simulink model "PGA_MPC_MODEL"  (R2024b)
settings: Solver=ode4  StartTime=0.0  StopTime=180  FixedStep=0.0005  RelTol=1e-3
values from neighbouring files (symbols this model uses):
  Road_Curvature_Map = [Global_S, Global_K]    [Road_Condition_Info.m]
  Road_Mu_Map = [Global_S, Global_Mu]    [Road_Condition_Info.m]
  Target_Speed_Map = [Global_S, Global_Vx]    [Road_Condition_Info.m]
undefined symbols (not defined in the file or in its folder): MotorData, Sim_Mu_Set, Sim_Vx_Set
libraries: Solver_SF x1
(part 2 of 3)

== matlab function PGA_MPC_MODEL/Subsystem1/MATLAB Function17 ==
  data: Vx input; r_d output; delta_f input; mu input; m input; lf input; lr input; K_s output; r_ideal output; Kf0 input; Kr0 input; g input; r_limit output
function [r_d, K_s, r_ideal, r_limit] = ReferenceYawRate(Vx, delta_f, mu, m, lf, lr, Kf0, Kr0, g)
% =========================================================================
% 参考横摆角速度生成 (鲁棒增强版)
% 修复内容：低速奇点保护、物理极限柔性化、输出平滑
% =========================================================================

    % 1. 参数默认值与保护
    if nargin < 9, g = 9.81; end
    
    % 输入数据维度清洗 (强制转为标量 double)
    Vx_in = double(Vx(1));
    delta_in = double(delta_f(1));
    mu_in = double(mu(1));

    % 速度方向与绝对值处理
    Vx_sign = sign(Vx_in);
    if Vx_sign == 0, Vx_sign = 1; end
    Vx_abs = abs(Vx_in);
    
    % 基础防除零保护 (计算模型用)
    Vx_safe = max(Vx_abs, 0.5); 

    % =====================================================================
    % 2. 计算稳态增益 (Steady State Gain)
    % =====================================================================
    K_s = m / (2 * (lf + lr)^2) * (lr/Kf0 - lf/Kr0);

    % =====================================================================
    % 3. 计算理想横摆角速度 (Linear 2DOF Model)
    % =====================================================================
    % 分母：1 + K * V^2
    denom = (lf + lr) * (1 + K_s * Vx_safe^2);
    
    if abs(denom) < 0.1
        r_ideal = 0;
    else
        % r_ideal = (Vx / L(1+KV^2)) * delta
        r_ideal = (Vx_safe / denom) * delta_in * Vx_sign; 
    end

    % =====================================================================
    % 4. 计算物理极限 (【关键修复点】)
    % =====================================================================
    % 原公式：Limit = 0.85 * mu * g / Vx
    % 问题：当车辆甩尾速度掉到 1m/s 时，Limit 会变成 0.85*0.8*9.8/1 = 6.6 rad/s (380度/秒)
    % 修复：计算极限时，假设速度至少为 5m/s (虚拟速度钳位)
    % 逻辑：低速时侧向加速度其实达不到 mu*g，因为离心力不够，所以这样限制更符合物理
    
    Vx_for_limit = max(Vx_abs, 5.0); 
    
    % 计算理论上限
    r_limit_val = 0.85 * mu_in * g / Vx_for_limit;
    
    % 【双重保险】增加一个绝对硬限幅 (例如 1.5 rad/s ≈ 85 deg/s)
    % 防止任何情况下的数值爆炸
    r_limit_val = min(r_limit_val, 1.5);

    % =====================================================================
    % 5. 柔性限幅 (Saturation)
    % =====================================================================
    if r_ideal > r_limit_val
        r_d_raw = r_limit_val;
    elseif r_ideal < -r_limit_val
        r_d_raw = -r_limit_val;
    else
        r_d_raw = r_ideal;
    end

    % =====================================================================
    % 6. 强力滤波 (平滑输出)
    % =====================================================================
    persistent rd_prev
    if isempty(rd_prev), rd_prev = 0; end
    
    % 滤波系数：0.05 代表非常强的滤波 (响应慢，但稳)，如果觉得滞后太大可改为 0.1
    alpha_filter = 0.05; 
    
    r_d_smooth = (1 - alpha_filter) * rd_prev + alpha_filter * r_d_raw;
    
    % 更新记忆
    rd_prev = r_d_smooth;

    % =====================================================================
    % 7. 输出类型转换
    % =====================================================================
    r_d = double(r_d_smooth);
    r_ideal = double(r_ideal);
    r_limit = double(r_limit_val);
    
end

== matlab function PGA_MPC_MODEL/Subsystem1/MATLAB Function15 ==
  data: Vx_cmd input; Vx_act_raw input; T_total output; Ax_cmd input; m input; g input; r_e input; Kp input; Ki input; dt input; is_reset input; T_ff output; T_fb output; delta_steering input; Mu_in input; Curv_in input; Beta_in input; SI_in input
function [T_total, T_ff, T_fb] = Calc_Total_Demand_Torque( ...
    Vx_cmd, Vx_act_raw, Ax_cmd, ...
    m, g, r_e, ...
    Kp, Ki, dt, is_reset, delta_steering, Mu_in, ...
    Curv_in, Beta_in, SI_in)
%#codegen
% =========================================================================
% Upper-layer nominal total torque generator v2
% 适配你的 H-MPC / AD-MPC 版本
%
% 核心原则：
%   1. 只负责生成“名义总需求转矩”
%   2. 不根据 Mu / Curv / Beta / SI 主动降扭
%   3. 不抢下层 MPC 的 Wsum 自适应调度功能
%   4. 自动处理 Vx_cmd 是 km/h 还是 m/s 的问题
%
% 推荐外部参数：
%   Kp = 12
%   Ki = 0.3
%   dt = 0.01
% =========================================================================

    persistent Vx_f I_term T_prev

    % =========================================================
    % 0. reset and basic protection
    % =========================================================
    reset_flag = false;
    if double(is_reset(1)) > 0.5
        reset_flag = true;
    end

    if dt <= 1e-6
        dt = 0.01;
    end

    Vx_cmd_raw = double(Vx_cmd(1));
    Vx_act_raw_use = double(Vx_act_raw(1));
    Ax_cmd_use = double(Ax_cmd(1));

    % =========================================================
    % 1. speed unit auto-detection
    % =========================================================
    % 你的工况是 68 km/h，CarSim Vx 通常约 18.9 m/s。
    % 如果输入大于 40，基本可以判断是 km/h，自动除以 3.6。
    if abs(Vx_cmd_raw) > 40.0
        Vx_cmd_use = Vx_cmd_raw / 3.6;
    else
        Vx_cmd_use = Vx_cmd_raw;
    end

    if abs(Vx_act_raw_use) > 40.0
        Vx_act_use = Vx_act_raw_use / 3.6;
    else
        Vx_act_use = Vx_act_raw_use;
    end

    Vx_cmd_use = max(0.0, Vx_cmd_use);
    Vx_act_use = max(0.0, Vx_act_use);

    if isempty(Vx_f) || reset_flag
        Vx_f   = Vx_act_use;
        I_term = 0.0;
        T_prev = 0.0;
    end

    % =========================================================
    % 2. actual speed filtering
    % =========================================================
    alpha_v = 0.15;
    Vx_f = (1.0 - alpha_v) * Vx_f + alpha_v * Vx_act_use;
    Vx_act = Vx_f;

    % =========================================================
    % 3. physical feedforward torque
    % =========================================================
    Cd = 0.30;
    Af = 2.8;
    rho = 1.206;
    f_roll = 0.015;

    Vx_ff = Vx_act;

    if abs(Vx_ff) > 0.2
        sgn_v = sign(Vx_ff);
    else
        sgn_v = 0.0;
    end

    % 不让 Ax_cmd 把上层变成激进加速器
    Ax_cmd_use = min(max(Ax_cmd_use, -0.8), 0.8);

    F_aero = 0.5 * rho * Cd * Af * Vx_ff * Vx_ff * sgn_v;
    F_roll = m * g * f_roll * sgn_v;
    F_acc  = m * Ax_cmd_use;

    T_ff = (F_aero + F_roll + F_acc) * r_e;

    % =========================================================
    % 4. mild PI speed feedback
    % =========================================================
    e_v = Vx_cmd_use - Vx_act;

    deadband = 0.08;

    if e_v > deadband
        e_eff = e_v - deadband;
    elseif e_v < -deadband
        e_eff = e_v + deadband;
    else
        e_eff = 0.0;
    end

    % 防止外部参数给太大
    Kp_eff = min(max(double(Kp), 0.0), 18.0);
    Ki_eff = min(max(double(Ki), 0.0), 1.0);

    P_term = Kp_eff * e_eff;

    % =========================================================
    % 5. integral with anti-windup
    % =========================================================
    I_max = 70.0;
    I_min = -90.0;

    I_candidate = I_term + Ki_eff * e_eff * dt;
    I_candidate = min(max(I_candidate, I_min), I_max);

    T_candidate = T_ff + P_term + I_candidate;

    % 名义总转矩保护，不根据风险变，只做物理合理范围限制
    T_max_limit = 320.0;
    T_min_limit = -180.0;

    if (T_candidate > T_max_limit && e_eff > 0.0)
        % 上限饱和且还想继续加速，不积分
    elseif (T_candidate < T_min_limit && e_eff < 0.0)
        % 下限饱和且还想继续减速，不积分
    else
        I_term = I_candidate;
    end

    T_cmd = T_ff + P_term + I_term;

    % =========================================================
    % 6. overspeed protection
    % =========================================================
    % 这不是稳定性控制，只是基本速度闭环保护：
    % 实际速度超过目标时，不允许上层继续大正转矩。
    over_v = Vx_act - Vx_cmd_use;

    if over_v > 0.25
        T_overspeed_limit = T_ff - 70.0 * over_v;
        T_cmd = min(T_cmd, T_overspeed_limit);
    end

    T_cmd = min(max(T_cmd, T_min_limit), T_max_limit);

    % =========================================================
    % 7. torque rate limit
    % =========================================================
    % 只做执行器平滑，不用风险信号。
    dT_up_rate = 350.0;    % Nm/s
    dT_dn_rate = 650.0;    % Nm/s

    dT_up = dT_up_rate * dt;
    dT_dn = dT_dn_rate * dt;

    if reset_flag
        T_total = T_cmd;
        T_prev = T_total;
    else
        dT = T_cmd - T_prev;

        if dT > dT_up
            T_total = T_prev + dT_up;
        elseif dT < -dT_dn
            T_total = T_prev - dT_dn;
        else
            T_total = T_cmd;
        end

        T_prev = T_total;
    end

    T_fb = T_total - T_ff;

    T_total = double(T_total);
    T_ff    = double(T_ff);
    T_fb    = double(T_fb);

end

== matlab function PGA_MPC_MODEL/Subsystem1/MATLAB Function18 ==
  settings: updateMethod=DISCRETE  sampleTime=0.01
  data: Vx_target_input input; Vx_safe_cmd output; dt input; Ax_cmd_final output
function [Vx_safe_cmd, Ax_cmd_final] = Constant_Speed_Planner(Vx_target_input, dt)
    % Constant_Speed_Planner
    % 功能：生成恒定目标车速和加速度指令
    
    % ================= 1. 数据预处理 (维度安全锁) =================
    % 强制转换为 double
    temp_v = double(Vx_target_input);
    
    % 【关键修改】防止输入变成向量 [4x1]
    % 如果输入是向量，取第一个元素或取平均值，确保输出是标量 [1x1]
    if numel(temp_v) > 1
        target_v = mean(temp_v); % 或者 target_v = temp_v(1);
    else
        target_v = temp_v;
    end
    
    % 限幅保护
    if isnan(target_v)
        target_v = 0;
    end
    target_v = max(target_v, 0); 

    % ================= 2. 指令生成 =================
    Vx_safe_cmd = target_v;
    
    % 理论加速度设为0
    Ax_cmd_final = 0; 
    
    % (可选) 如果未来想用 dt 做平滑处理，可以在这里写逻辑
    % 目前 dt 虽然未被使用，但保留在输入端口没问题，不会报错
end

== matlab function PGA_MPC_MODEL/Subsystem1/MATLAB Function19 ==
  data: Vx input; Beta input; Beta_dot input; mu input; SI_Out output
function SI_Out = fcn_Calculate_SI(Vx, Beta, Beta_dot, mu)
%#codegen
% =========================================================================
% SI calculation module without upper saturation
% Purpose:
%   Used for post-processing, logging, and quantitative comparison.
%   The upper bound of 1.5 is removed so that the true instability severity
%   can be observed in simulation results.
% =========================================================================

    %% 1. Input processing
    v_in = max(abs(double(Vx(1))), 1.0);
    beta_in = double(Beta(1));
    beta_dot_in = double(Beta_dot(1));
    mu_in = max(min(double(mu(1)), 0.9), 0.2);

    %% 2. Phase-plane boundary slope
    % Slope = -0.000005 * v^2 + 0.003898 * v + 0.022393
    Slope = -0.000005 * v_in^2 + 0.003898 * v_in + 0.022393;

    %% 3. Stability boundary Blim
    e1 = -0.038102; 
    e2 =  0.195963; 
    e3 =  0.005132;
    e4 =  0.235299; 
    e5 = -0.011306; 
    e6 = -0.000252;
    e7 = -0.013729; 
    e8 =  0.000720; 
    e9 = -0.000046;

    Blim = e1 + ...
           e2 * mu_in + e3 * v_in + ...
           e4 * mu_in^2 + e5 * mu_in * v_in + e6 * v_in^2 + ...
           e7 * mu_in^2 * v_in + e8 * mu_in * v_in^2 + ...
           e9 * mu_in^2 * v_in^2;

    % Boundary protection
    if Blim < 0.001
        Blim = 0.001;
    end

    %% 4. SI calculation
    % Stability boundary:
    % | beta + Slope * beta_dot | <= Blim
    Phase_Val = beta_in + Slope * beta_dot_in;
    SI_phase = abs(Phase_Val) / abs(Blim);

    %% 5. Physical fallback
    % If sideslip angle exceeds about 10 deg, the vehicle is regarded as
    % approaching severe instability.
    SI_Phys = abs(beta_in) / 0.17;

    %% 6. Final SI output without upper saturation
    SI_Out = max(SI_phase, SI_Phys);

    % Keep only the lower bound protection. No upper saturation is applied.
    SI_Out = max(SI_Out, 0);
end

== matlab function PGA_MPC_MODEL/Subsystem1/MATLAB Function23 ==
  data: Fy_fl input; Cf_eq output; Fy_fr input; Fy_rl input; Fy_rr input; Alpha_fl input; Alpha_fr input; Alpha_rl input; Alpha_rr input; Cf0 input; Cr0 input; Cr_eq output; Mu_Current input
function [Cf_eq, Cr_eq] = fcn_Calc_Equivalent_Stiffness_Filtered(...
    Fy_fl, Fy_fr, Fy_rl, Fy_rr, ...
    Alpha_fl, Alpha_fr, Alpha_rl, Alpha_rr, ...
    Cf0, Cr0, Mu_Current) % ★ 新增输入: 当前路面附着 Mu_Current
% =========================================================================
% 非线性侧偏刚度估算模块 (前馈预警 + 实时估算混合版)
% =========================================================================
    persistent Cf_prev Cr_prev
    if isempty(Cf_prev)
        Cf_prev = Cf0 * 2; 
        Cr_prev = Cr0 * 2;
    end
    
    % =====================================================================
    % ★ 核心新增：基于附着系数的前馈压制 (Feed-forward Penalty) ★
    % 当车进入冰雪路面时，不用等侧滑发生，直接从物理极限上压低标称刚度！
    % =====================================================================
    mu_nominal = 0.85;
    mu_real = max(min(double(Mu_Current(1)), 1.0), 0.1);
    % 计算附着衰减系数
    mu_ratio = mu_real / mu_nominal; 
    
    % 前馈修正后的基础刚度 (冰面上基础刚度会瞬间掉下来)
    Cf_base_dyn = (Cf0 * 2) * mu_ratio;
    Cr_base_dyn = (Cr0 * 2) * mu_ratio;

    Fy_front_sum = abs(Fy_fl + Fy_fr);
    Fy_rear_sum  = abs(Fy_rl + Fy_rr);
    Alpha_front_avg = abs(Alpha_fl + Alpha_fr) / 2.0;
    Alpha_rear_avg  = abs(Alpha_rl + Alpha_rr) / 2.0;
    
    alpha_deadzone = 0.0087; 
    
    if Alpha_front_avg > alpha_deadzone
        Cf_inst = Fy_front_sum / Alpha_front_avg;
    else
        Cf_inst = Cf_base_dyn; % 小角度时用前馈修正的刚度
    end
    
    if Alpha_rear_avg > alpha_deadzone
        Cr_inst = Fy_rear_sum / Alpha_rear_avg;
    else
        Cr_inst = Cr_base_dyn; % 小角度时用前馈修正的刚度
    end
    
    % ★ 限幅逻辑也要跟着附着系数前馈一起下降 ★
    Cf_min = Cf_base_dyn * 0.3;  Cf_max = Cf_base_dyn * 1.5;
    Cr_min = Cr_base_dyn * 0.3;  Cr_max = Cr_base_dyn * 1.5;
    
    Cf_target = max(min(Cf_inst, Cf_max), Cf_min);
    Cr_target = max(min(Cr_inst, Cr_max), Cr_min);
    
    % 为了应对附着突变，如果是从高附着到低附着（刚度需要暴降），加快滤波速度
    if Cf_target < Cf_prev
        lambda = 0.3; % 变滑了，降刚度要快！(0.05太慢了)
    else
        lambda = 0.05; % 恢复抓地力，慢慢升
    end
    
    Cf_filt = (1 - lambda) * Cf_prev + lambda * Cf_target;
    Cr_filt = (1 - lambda) * Cr_prev + lambda * Cr_target;
    
    Cf_prev = Cf_filt; Cr_prev = Cr_filt;
    Cf_eq = Cf_filt; Cr_eq = Cr_filt;
end

== matlab function PGA_MPC_MODEL/Subsystem1/MATLAB Function5 ==
  data: Vx input; Sx_fr output; Vy input; r input; omega_fr input; delta_f input; lf input; twf input; Re input; Sy_fr output; Vsx_fr output; Vsy_fr output
function [Sx_fr, Sy_fr, Vsx_fr, Vsy_fr] = Cal_UniTire_FullData_FR(Vx, Vy, r, omega_fr, delta_f, lf, twf, Re)
% Cal_UniTire_FullData_FR - 右前轮全参数计算

    % === 1. 运动学解算 ===
    % 右前轮：纵向 +lf, 横向 -twf/2 (右侧)
    % Vx修正: 右侧轮在左转(r>0)时线速度增加，所以是 + r*(twf/2)
    V_cx = Vx + r * (twf / 2);  
    V_cy = Vy + r * lf;         

    % === 2. 坐标旋转 (车轮坐标系) ===
    cos_d = cos(delta_f);
    sin_d = sin(delta_f);
    
    V_long = V_cx * cos_d + V_cy * sin_d;
    V_lat  = -V_cx * sin_d + V_cy * cos_d;

    % === 3. 计算滑移速度 (能耗用) ===
    V_wheel = omega_fr * Re;
    Vsx_fr = V_wheel - V_long; % 纵向滑移速度
    Vsy_fr = V_lat;            % 侧向滑移速度

    % === 4. 计算滑移率 (轮胎模型用) ===
    V_long_safe = max(abs(V_long), 1.0); 
    
    Sx_fr = Vsx_fr / V_long_safe;
    Sy_fr = -Vsy_fr / V_long_safe; % UniTire定义带负号

    % === 5. 限幅 ===
    Sx_fr = max(min(Sx_fr, 1.5), -1.5);
    Sy_fr = max(min(Sy_fr, 1.5), -1.5);
end

== matlab function PGA_MPC_MODEL/Subsystem1/MATLAB Function6 ==
  data: Vx input; Sx_rl output; Vy input; r input; omega_rl input; lr input; twr input; Re input; Sy_rl output; Vsx_rl output; Vsy_rl output
function [Sx_rl, Sy_rl, Vsx_rl, Vsy_rl] = Cal_UniTire_FullData_RL(Vx, Vy, r, omega_rl, lr, twr, Re)
% Cal_UniTire_FullData_RL - 左后轮全参数计算
% 注意：后轮默认无转向角 (delta = 0)

    % === 1. 运动学解算 ===
    % 左后轮：纵向 -lr, 横向 +twr/2 (左侧)
    % Vcx: 左侧减去横摆分量
    % Vcy: 后轴减去横摆分量 (Vy - r*lr)
    V_cx = Vx - r * (twr / 2);  
    V_cy = Vy - r * lr;         

    % === 2. 坐标旋转 (后轮 delta=0) ===
    % cos(0)=1, sin(0)=0，其实就是不用旋转
    V_long = V_cx;
    V_lat  = V_cy;

    % === 3. 计算滑移速度 (能耗用) ===
    V_wheel = omega_rl * Re;
    Vsx_rl = V_wheel - V_long; 
    Vsy_rl = V_lat;            

    % === 4. 计算滑移率 (轮胎模型用) ===
    V_long_safe = max(abs(V_long), 1.0); 
    
    Sx_rl = Vsx_rl / V_long_safe;
    Sy_rl = -Vsy_rl / V_long_safe;

    % === 5. 限幅 ===
    Sx_rl = max(min(Sx_rl, 1.5), -1.5);
    Sy_rl = max(min(Sy_rl, 1.5), -1.5);
end

== matlab function PGA_MPC_MODEL/Subsystem1/MATLAB Function7 ==
  data: Vx input; Sx_rr output; Vy input; r input; omega_rr input; lr input; twr input; Re input; Sy_rr output; Vsx_rr output; Vsy_rr output
function [Sx_rr, Sy_rr, Vsx_rr, Vsy_rr] = Cal_UniTire_FullData_RR(Vx, Vy, r, omega_rr, lr, twr, Re)
% Cal_UniTire_FullData_RR - 右后轮全参数计算
% 注意：后轮默认无转向角 (delta = 0)

    % === 1. 运动学解算 ===
    % 右后轮：纵向 -lr, 横向 -twr/2 (右侧)
    % Vcx: 右侧加上横摆分量
    % Vcy: 后轴减去横摆分量
    V_cx = Vx + r * (twr / 2);  
    V_cy = Vy - r * lr;         

    % === 2. 坐标旋转 (后轮 delta=0) ===
    V_long = V_cx;
    V_lat  = V_cy;

    % === 3. 计算滑移速度 (能耗用) ===
    V_wheel = omega_rr * Re;
    Vsx_rr = V_wheel - V_long; 
    Vsy_rr = V_lat;            

    % === 4. 计算滑移率 (轮胎模型用) ===
    V_long_safe = max(abs(V_long), 1.0); 
    
    Sx_rr = Vsx_rr / V_long_safe;
    Sy_rr = -Vsy_rr / V_long_safe;

    % === 5. 限幅 ===
    Sx_rr = max(min(Sx_rr, 1.5), -1.5);
    Sy_rr = max(min(Sy_rr, 1.5), -1.5);
end

== matlab function PGA_MPC_MODEL/Subsystem1/unitire轮胎力 ==
  data: Vx input; Vy input; r input; Sx_fl output; omega_fl input; delta_f input; lf input; twf input; Sy_fl output; Re input; Vsx_fl output; Vsy_fl output
function [Sx_fl, Sy_fl, Vsx_fl, Vsy_fl] = Cal_UniTire_FullData_FL(Vx, Vy, r, omega_fl, delta_f, lf, twf, Re)
% Cal_UniTire_FullData_FL - 左前轮全参数计算
% 输出: 
%   Sx, Sy: UniTire定义的滑移率 (无量纲) -> 用于查表或公式算力
%   Vsx, Vsy: 轮胎接地点滑移速度 (m/s) -> 用于 P = F * V 算能耗

    % === 1. 运动学解算：计算【轮心】在【车身坐标系】下的速度 ===
    % (左前轮：纵向 +lf, 横向 +twf/2)
    % 注意：横摆 r 对纵向速度的影响是 -r*y, 对横向速度的影响是 +r*x
    V_cx = Vx - r * (twf / 2);  
    V_cy = Vy + r * lf;         

    % === 2. 坐标旋转：转换到【车轮坐标系】 ===
    cos_d = cos(delta_f);
    sin_d = sin(delta_f);
    
    % V_long: 车轮滚动方向速度 (即纵向速度 Vx_wheel)
    % V_lat:  车轮侧向速度 (即侧向速度 Vy_wheel)
    V_long = V_cx * cos_d + V_cy * sin_d;
    V_lat  = -V_cx * sin_d + V_cy * cos_d;

    % === 3. 计算滑移速度 (能耗计算的核心) ===
    % 轮缘线速度
    V_wheel = omega_fl * Re;

    % 纵向滑移速度 (Vsx): 也就是大家常说的“滑移速度差”
    % 物理含义：轮胎接地点相对于地面的向后速度
    Vsx_fl = V_wheel - V_long; 

    % 侧向滑移速度 (Vsy): 
    % 物理含义：轮胎整体侧滑的速度
    Vsy_fl = V_lat; 

    % === 4. 计算滑移率 (UniTire 轮胎力模型的核心) ===
    % 分母保护：防止停车或低速时除零，导致仿真崩溃
    % 选取 max(abs(V_long), 1.0) 是为了在低速下保证数值稳定
    V_long_safe = max(abs(V_long), 1.0); 
    
    % --- 纵向滑移率 Sx ---
    % UniTire 定义: Sx = (V_wheel - V_long) / V_long
    % 等价于: Sx = Vsx / V_long
    Sx_fl = Vsx_fl / V_long_safe;

    % --- 侧向滑移率 Sy ---
    % UniTire 定义: Sy = - V_lat / V_long
    % 等价于: Sy = - Vsy / V_long
    % 注意：UniTire 的 Sy 定义通常带有负号 (对应 -tan(alpha))
    Sy_fl = -Vsy_fl / V_long_safe;

    % === 5. 物理限幅 (防止数值爆炸) ===
    % 仅对滑移率限幅，滑移速度(Vsx/Vsy)是物理真值，不要限幅！
    Sx_fl = max(min(Sx_fl, 1.5), -1.5);
    Sy_fl = max(min(Sy_fl, 1.5), -1.5);

end

== matlab function PGA_MPC_MODEL/Subsystem1/侧偏角计算 ==
  data: Vx input; alpha_fl output; Vy input; r input; delta_f_rad input; lf input; lr input; twf input; twr input; alpha_fr output; alpha_rl output; alpha_rr output
function [alpha_fl, alpha_fr, alpha_rl, alpha_rr] = Block2_SlipAngle(...
    Vx, Vy, r, delta_f_rad, lf, lr, twf, twr)
% =========================================================================
% BLOCK2_SLIPANGLE - 四轮侧偏角计算 (纯弧度版)
% 
% [关键设置]
% 1. 输入 delta_f_rad 必须是【弧度】(您已在外部转换好)。
% 2. 输出 alpha 均为【弧度】。
% 3. 符号修正：采用 (转向角 - 速度角) 逻辑，确保左转产生正滑移角。
% =========================================================================

    % 1. 速度方向保护 (防止分母为0)
    Vx_safe = max(abs(Vx), 0.1) * sign(Vx); 
    if Vx_safe == 0, Vx_safe = 0.1; end
    
    % 2. 轮心速度解算 (运动学公式)
    % -----------------------------------------------------------
    % 左前轮 (Left-Front)
    Vx_fl = Vx_safe - (r * twf) / 2;
    Vy_fl = Vy + (r * lf);
    
    % 右前轮 (Right-Front)
    Vx_fr = Vx_safe + (r * twf) / 2;
    Vy_fr = Vy + (r * lf);
    
    % 左后轮 (Left-Rear)
    Vx_rl = Vx_safe - (r * twr) / 2;
    Vy_rl = Vy - (r * lr);
    
    % 右后轮 (Right-Rear)
    Vx_rr = Vx_safe + (r * twr) / 2;
    Vy_rr = Vy - (r * lr);
    
    % 3. 侧偏角计算 (核心修正)
    % -----------------------------------------------------------
    % 公式：Alpha = 转向角 - 速度矢量角
    % atan2 计算结果天然是弧度，与您的输入 delta_f_rad (弧度) 直接相减
    
    % 左前
    theta_fl = atan2(Vy_fl, Vx_fl);
    alpha_fl = delta_f_rad - theta_fl; 
    
    % 右前
    theta_fr = atan2(Vy_fr, Vx_fr);
    alpha_fr = delta_f_rad - theta_fr;
    
    % 左后 (后轮转向角 delta = 0)
    theta_rl = atan2(Vy_rl, Vx_rl);
    alpha_rl = 0 - theta_rl; 
    
    % 右后
    theta_rr = atan2(Vy_rr, Vx_rr);
    alpha_rr = 0 - theta_rr; 

    % 4. 输出清理
    % -----------------------------------------------------------
    % 确保输出为实数
    alpha_fl = real(alpha_fl);
    alpha_fr = real(alpha_fr);
    alpha_rl = real(alpha_rl);
    alpha_rr = real(alpha_rr);
    
    % [注意] 输出的是弧度！
    % 如果接下来的刚度模块或轮胎模块需要弧度，直接连线即可。
    % 后面【千万不要】再接那个 pi/180 的 Gain 模块了！
end

== matlab function PGA_MPC_MODEL/Subsystem1/横纵向附着系数 ==
  data: road_condition input; mu_x output; slip_ratio input; mu_y output
function [mu_x, mu_y] = FrictionCoefficientLookup(road_condition, slip_ratio)
% 基于路面条件和滑移率的摩擦系数查表
% 输入: road_condition - 路面类型 (1=冰面, 2=雪面, 3=湿沥青, 4=干沥青)
%       slip_ratio - 当前滑移率（可选，用于动态调整）

    switch road_condition
        case 1 % 冰面（论文实验条件）
            mu_x = 0.2;
            mu_y = 0.18;  % 横向摩擦系数通常略低
            
        case 2 % 雪面
            mu_x = 0.3;
            mu_y = 0.25;
            
        case 3 % 湿沥青
            mu_x = 0.5;
            mu_y = 0.45;
            
        case 4 % 干沥青
            mu_x = 0.85;
            mu_y = 0.80;
            
        otherwise
            mu_x = 0.8;
            mu_y = 0.75;
    end
    
    % 可选：基于滑移率的动态调整（Burckhardt模型简化版）
    if nargin > 1
        % 典型摩擦系数-滑移率曲线（冰面）
        if road_condition == 1
            optimal_slip = 0.08;  % 冰面最佳滑移率
            if slip_ratio > optimal_slip
                % 超过最佳滑移率后摩擦系数下降
                mu_x = mu_x * (1 - 0.5 * (slip_ratio - optimal_slip));
                mu_y = mu_y * (1 - 0.6 * (slip_ratio - optimal_slip));
            end
        end
    end
end

== matlab function PGA_MPC_MODEL/Subsystem1/MATLAB Function1 ==
  data: Sx_fl input; Sy_fl input; Fx_fl output; Fz_fl input; mu_x input; mu_y input; Kx input; Ky input; Fy_fl output; Fbar_x_fl output; Fbar_y_fl output; E input
function [Fx_fl, Fy_fl, Fbar_x_fl, Fbar_y_fl] = Cal_Force_FL(Sx_fl, Sy_fl, Fz_fl, mu_x, mu_y, Kx, Ky, E)
% Cal_Force_FL - 左前轮 UniTire (完整版)
% 输入:
% Sx_fl, Sy_fl: 纵横向滑移率
% Fz_fl: 垂向载荷 (N)
% mu_x, mu_y: 纵向/横向 峰值附着系数 (例如 1.0, 0.9)
% Kx, Ky: 轮胎纵向/横向刚度 (N/1)
% E: UniTire 曲率因子 (通常 0.5~1.0，决定峰值后的形状)

% 0. 数据保护
Fz_safe = max(Fz_fl, 100); % 防止 Fz=0 报错
% 1. 计算相对滑移率 (Relative Slip, phi)
% 分别针对纵向和横向极限进行归一化
% phi_x = (Kx * Sx) / (mu_x * Fz)
phi_x = (Kx * abs(Sx_fl)) / (mu_x * Fz_safe);
phi_y = (Ky * abs(Sy_fl)) / (mu_y * Fz_safe);
% 合成相对滑移率 (摩擦椭圆耦合核心)
phi = sqrt(phi_x^2 + phi_y^2);

% 2. 计算总归一化力 (F_bar)
% UniTire 经验公式: F_bar = 1 - exp(-phi - E * phi^2)
% 这里的 E 就是您要找回的曲率因子
if phi < 1e-6
F_bar = 0;
else
F_bar = 1 - exp(-phi - E * phi^2);
end

% 3. 分解回横纵向 (分配方向)
% Fbar_x 是归一化分量 (0~1)
if phi < 1e-6
Fbar_x_fl = 0;
Fbar_y_fl = 0;
else
Fbar_x_fl = F_bar * (phi_x / phi);
Fbar_y_fl = F_bar * (phi_y / phi);
end

% 4. 计算真实物理力 (Physical Force, N)
% 必须乘回各自方向的极限力 (mu * Fz)
Max_Force_X = mu_x * Fz_safe;
Max_Force_Y = mu_y * Fz_safe;
Fx_abs = Fbar_x_fl * Max_Force_X;
Fy_abs = Fbar_y_fl * Max_Force_Y;

% 5. 恢复符号
Fx_fl = sign(Sx_fl) * Fx_abs;
Fy_fl = sign(Sy_fl) * Fy_abs;
end

== matlab function PGA_MPC_MODEL/Subsystem1/MATLAB Function8 ==
  data: Sx_rl input; Sy_rl input; Fx_rl output; Fz_rl input; mu_x input; mu_y input; Kx input; Ky input; Fy_rl output; Fbar_x_rl output; Fbar_y_rl output; E input

function [Fx_rl, Fy_rl, Fbar_x_rl, Fbar_y_rl] = Cal_Force_RL(Sx_rl, Sy_rl, Fz_rl, mu_x, mu_y, Kx, Ky, E)
% Cal_Force_RL - 左后轮 UniTire (完整版)

Fz_safe = max(Fz_rl, 100);

% 1. 相对滑移率
phi_x = (Kx * abs(Sx_rl)) / (mu_x * Fz_safe);
phi_y = (Ky * abs(Sy_rl)) / (mu_y * Fz_safe);
phi = sqrt(phi_x^2 + phi_y^2);

% 2. 总归一化力
if phi < 1e-6
F_bar = 0;
else
F_bar = 1 - exp(-phi - E * phi^2);
end

% 3. 分量分配
if phi < 1e-6
Fbar_x_rl = 0;
Fbar_y_rl = 0;
else
Fbar_x_rl = F_bar * (phi_x / phi);
Fbar_y_rl = F_bar * (phi_y / phi);
end

% 4. 真实力
Fx_rl = sign(Sx_rl) * (Fbar_x_rl * (mu_x * Fz_safe));
Fy_rl = sign(Sy_rl) * (Fbar_y_rl * (mu_y * Fz_safe));
end

== matlab function PGA_MPC_MODEL/Subsystem1/MATLAB Function9 ==
  data: Sx_fr input; Sy_fr input; Fx_fr output; Fz_fr input; mu_x input; mu_y input; Kx input; Ky input; Fy_fr output; Fbar_x_fr output; Fbar_y_fr output; E input
function [Fx_fr, Fy_fr, Fbar_x_fr, Fbar_y_fr] = Cal_Force_FR(Sx_fr, Sy_fr, Fz_fr, mu_x, mu_y, Kx, Ky, E)
% Cal_Force_FR - 右前轮 UniTire (完整版)

Fz_safe = max(Fz_fr, 100);

% 1. 相对滑移率
phi_x = (Kx * abs(Sx_fr)) / (mu_x * Fz_safe);
phi_y = (Ky * abs(Sy_fr)) / (mu_y * Fz_safe);
phi = sqrt(phi_x^2 + phi_y^2);

% 2. 总归一化力 (带 E)
if phi < 1e-6
F_bar = 0;
else
F_bar = 1 - exp(-phi - E * phi^2);
end

% 3. 分量分配
if phi < 1e-6
Fbar_x_fr = 0;
Fbar_y_fr = 0;
else
Fbar_x_fr = F_bar * (phi_x / phi);
Fbar_y_fr = F_bar * (phi_y / phi);
end

% 4. 真实力 (乘回 mu*Fz)
Fx_fr = sign(Sx_fr) * (Fbar_x_fr * (mu_x * Fz_safe));
Fy_fr = sign(Sy_fr) * (Fbar_y_fr * (mu_y * Fz_safe));
end

== matlab function PGA_MPC_MODEL/Subsystem1/MATLAB Function10 ==
  data: Sx_rr input; Sy_rr input; Fx_rr output; Fz_rr input; mu_x input; mu_y input; Kx input; Ky input; E input; Fy_rr output; Fbar_x_rr output; Fbar_y_rr output
function [Fx_rr, Fy_rr, Fbar_x_rr, Fbar_y_rr] = Cal_Force_RR(Sx_rr, Sy_rr, Fz_rr, mu_x, mu_y, Kx, Ky, E)
% Cal_Force_RR - 右后轮 UniTire (完整版)

Fz_safe = max(Fz_rr, 100);

% 1. 相对滑移率
phi_x = (Kx * abs(Sx_rr)) / (mu_x * Fz_safe);
phi_y = (Ky * abs(Sy_rr)) / (mu_y * Fz_safe);
phi = sqrt(phi_x^2 + phi_y^2);

% 2. 总归一化力
if phi < 1e-6
F_bar = 0;
else
F_bar = 1 - exp(-phi - E * phi^2);
end

% 3. 分量分配
if phi < 1e-6
Fbar_x_rr = 0;
Fbar_y_rr = 0;
else
Fbar_x_rr = F_bar * (phi_x / phi);
Fbar_y_rr = F_bar * (phi_y / phi);
end

% 4. 真实力
Fx_rr = sign(Sx_rr) * (Fbar_x_rr * (mu_x * Fz_safe));
Fy_rr = sign(Sy_rr) * (Fbar_y_rr * (mu_y * Fz_safe));
end

== matlab function PGA_MPC_MODEL/Subsystem1/MATLAB Function14 ==
  data: NN_Weights output; Vx_kmh input; Vref_kmh input; Mu_current input; Kappa_current input; Mu_preview input; Kappa_preview input
function NN_Weights = Call_NN_Mapper(Vx_kmh, Vref_kmh, Mu_current, Kappa_current, Mu_preview, Kappa_preview)
%#codegen
% =========================================================================
% Reference-speed-aware risk-preserving 4D BO-BPNN weight mapper
%
% BPNN input:
%   X_NN = [V_NN, mu_risk, kappa_risk, D_safe]^T
%
% Key idea:
%   1) The BPNN still uses a 4D input.
%   2) The first input is not the raw measured speed, but a risk-preserving
%      speed feature V_NN.
%   3) In low-risk conditions, V_NN follows the measured speed Vx.
%   4) In high-risk conditions, V_NN approaches the reference-speed-aware
%      risk speed, but is capped to avoid excessive conservativeness.
% =========================================================================

    NN_Weights = zeros(5, 1, 'double');

    %% ============================================================
    % 0. Tunable parameters
    % ============================================================
    Ts_ctrl = 0.01;          % Control sampling time, s

    D_low  = 0.50;           % Risk-gate lower threshold
    D_high = 0.70;           % Risk-gate upper threshold

    DeltaV_cap = 10.0;        % km/h, max allowed gap between V_NN and Vx
                             % If SI is still high, try 10~12.
                             % If speed drops too much, try 5~6.

    lambda_D = 0.10;         % 1/s, linear decay rate of D_safe

    %% ============================================================
    % 1. Signal reading and protection
    % ============================================================
    Vx = double(Vx_kmh(1));
    if ~isfinite(Vx)
        Vx = 60.0;
    end
    Vx = min(max(Vx, 0.0), 120.0);

    Vref = double(Vref_kmh(1));
    if ~isfinite(Vref) || Vref <= 1.0
        Vref = Vx;
    end
    Vref = min(max(Vref, 0.0), 120.0);

    Mu_c = double(Mu_current(1));
    Mu_p = double(Mu_preview(1));

    if ~isfinite(Mu_c) || Mu_c <= 0
        Mu_c = 0.85;
    end

    if ~isfinite(Mu_p) || Mu_p <= 0
        Mu_p = Mu_c;
    end

    mu_risk = min(Mu_c, Mu_p);
    mu_risk = max(mu_risk, 0.10);

    Kappa_c = abs(double(Kappa_current(1)));
    Kappa_p = abs(double(Kappa_preview(1)));

    if ~isfinite(Kappa_c)
        Kappa_c = 0.0;
    end

    if ~isfinite(Kappa_p)
        Kappa_p = 0.0;
    end

    kappa_risk = max(Kappa_c, Kappa_p);

    %% ============================================================
    % 2. Reference-speed-aware risk gate
    % ============================================================
    D_ref = ((Vref / 3.6)^2 * kappa_risk) / max(mu_risk * 9.81, 1e-6);
    D_ref = min(max(D_ref, 0.0), 1.0);

    gamma = (D_ref - D_low) / max(D_high - D_low, 1e-6);
    gamma = min(max(gamma, 0.0), 1.0);

    %% ============================================================
    % 3. Risk-preserving speed feature
    % ============================================================
    V_risk = min(Vref, Vx + DeltaV_cap);
    V_risk = max(V_risk, Vx);

    V_NN = (1.0 - gamma) * Vx + gamma * V_risk;
    V_NN = min(max(V_NN, 0.0), 120.0);

    %% ============================================================
    % 4. Risk calculation with linear peak-hold decay
    % ============================================================
    D_raw = ((V_NN / 3.6)^2 * kappa_risk) / max(mu_risk * 9.81, 1e-6);
    D_raw = min(max(D_raw, 0.0), 1.0);

    persistent D_safe_prev;
    if isempty(D_safe_prev)
        D_safe_prev = 0.0;
    end

    D_safe = max(D_raw, D_safe_prev - lambda_D * Ts_ctrl);
    D_safe = min(max(D_safe, 0.0), 1.0);
    D_safe_prev = D_safe;

    %% ============================================================
    % 5. BPNN forward inference
    % ============================================================
    X_in = [V_NN; mu_risk; kappa_risk; D_safe];

    NN_out = BPNN_Core_Ultimate_Res(X_in);

    %% ============================================================
    % 6. Physical baseline and NN residual reconstruction
    % ============================================================
    base_R = 4.5 - 3.5 * D_safe;
    base_W = 1.0 + 3.5 * D_safe;

    res_R_alloc = max(-2.0, min(2.0, NN_out(3)));
    res_W_slip  = max(-2.0, min(3.0, NN_out(5)));

    log_R_alloc_nn = base_R + res_R_alloc;
    log_W_slip_nn  = base_W + res_W_slip;

    log_Q_beta_nn = NN_out(1);
    log_Q_yaw_nn  = NN_out(2);
    log_R_rate_nn = NN_out(4) - 0.5 * (D_safe^2);

    %% ============================================================
    % 7. Risk-dependent safety envelope for W_slip
    % ============================================================
    envelope_W = -16.2 * (D_safe^2) + 32.8 * D_safe - 11.6;
    envelope_W = max(0.0, envelope_W);

    log_W_slip_final = max(log_W_slip_nn, envelope_W);

    %% ============================================================
    % 8. High-risk priority shift
    % ============================================================
    risk_barrier = max(0.0, D_safe - 0.7) / 0.3;
    risk_barrier = min(max(risk_barrier, 0.0), 1.0);

    penalty_others = 1.0 * risk_barrier;

    log_R_alloc_final = log_R_alloc_nn - penalty_others;
    log_R_rate_final  = log_R_rate_nn  - penalty_others;
    log_Q_beta_final  = log_Q_beta_nn  - penalty_others;
    log_Q_yaw_final   = log_Q_yaw_nn   - penalty_others;

    %% ============================================================
    % 9. Log-domain bounds
    % ============================================================
    log_W_slip_final  = max(-1.0, min(5.5, log_W_slip_final));
    log_R_alloc_final = max(-1.0, min(6.0, log_R_alloc_final));
    log_R_rate_final  = max(-1.0, min(6.0, log_R_rate_final));
    log_Q_beta_final  = max(-1.0, min(6.0, log_Q_beta_final));
    log_Q_yaw_final   = max(-1.0, min(6.0, log_Q_yaw_final));

    %% ============================================================
    % 10. Log-domain filtering
    % ============================================================
    logW_raw = [
        log_Q_beta_final;
        log_Q_yaw_final;
        log_R_alloc_final;
        log_R_rate_final;
        log_W_slip_final
    ];

    persistent logW_prev;
    if isempty(logW_prev)
        logW_prev = logW_raw;
    end

    alpha = 0.1 + 0.3 * D_safe;
    alpha = min(max(alpha, 0.05), 0.45);

    logW_filt = (1.0 - alpha) * logW_prev + alpha * logW_raw;
    logW_prev = logW_filt;

    %% ============================================================
    % 11. Exponential reconstruction
    % ============================================================
    NN_Weights(1) = 10^logW_filt(1);   % Q_beta
    NN_Weights(2) = 10^logW_filt(2);   % Q_r
    NN_Weights(3) = 10^logW_filt(3);   % R_alloc
    NN_Weights(4) = 10^logW_filt(4);   % R_rate
    NN_Weights(5) = 10^logW_filt(5);   % W_slip
end

== matlab function PGA_MPC_MODEL/Subsystem1/MATLAB Function16 ==
  data: Fx_fl input; Px_fl output; Fy_fl input; Sx_fl input; Sy_fl input; Vx input; Vy input; r input; delta_f input; lf input; twf input; Py_fl output
function [Px_fl, Py_fl] = Cal_Power_FL(Fx_fl, Fy_fl, Sx_fl, Sy_fl, Vx, Vy, r, delta_f, lf, twf)
% Cal_Power_FL - 左前轮横纵向滑移功耗计算
% 基于 UniTire 模型定义的滑移率和力进行能量损耗计算
%
% 输入:
%   Fx_fl, Fy_fl: 轮胎纵向/横向力 (N) [来自力计算模块]
%   Sx_fl, Sy_fl: 轮胎纵向/横向滑移率 [来自滑移率模块]
%   Vx, Vy: 质心速度 (m/s)
%   r: 横摆角速度 (rad/s)
%   delta_f: 前轮转角 (rad)
%   lf: 质心到前轴距离 (m)
%   twf: 前轮距 (m)
%
% 输出:
%   Px_fl: 纵向滑移功耗 (W)
%   Py_fl: 横向滑移功耗 (W)

    % 1. 重新计算轮心纵向速度 V_long (用于将滑移率还原为滑移速度)
    % 运动学：左前轮位置 (+lf, +twf/2)
    V_cx = Vx - r * (twf / 2); % 减去横摆线速度
    V_cy = Vy + r * lf;        % 加上横摆线速度

    % 坐标旋转到车轮坐标系
    cos_d = cos(delta_f);
    sin_d = sin(delta_f);
    
    % V_long 是车轮滚动方向的速度
    V_long = V_cx * cos_d + V_cy * sin_d;
    
    % 保护：防止低速除零或噪声，与滑移率模块保持一致的基准
    V_long_abs = max(abs(V_long), 1.0);

    % 2. 计算纵向滑移功耗 (Longitudinal Slip Power)
    % 公式: Power = Force * Sliding_Velocity
    % Sliding_Velocity_X = Sx * V_long
    % 取绝对值因为功耗总是正值 (能量耗散)
    Px_fl = abs(Fx_fl * (Sx_fl * V_long_abs));

    % 3. 计算横向滑移功耗 (Lateral Slip Power)
    % 公式: Power = Force * Lateral_Sliding_Velocity
    % 根据 UniTire 定义: Sy = -V_lat / V_long  => V_lat = -Sy * V_long
    % 同样取绝对值
    Py_fl = abs(Fy_fl * (Sy_fl * V_long_abs));

end

== matlab function PGA_MPC_MODEL/Subsystem1/MATLAB Function21 ==
  data: Fx input; E_long_J output; E_lat_J output; Fy input; Vsx input; Vsy input; dt input; is_reset input; E_slip_J output; E_slip_kWh output; P_long_W output; P_lat_W output
function [E_long_J, E_lat_J, E_slip_J, E_slip_kWh, P_long_W, P_lat_W] = ...
    Cal_Slip_Energy_Internal_v2(Fx, Fy, Vsx, Vsy, dt, is_reset)
%#codegen
% =========================================================================
% Tire slip dissipation calculation
%
% Fx, Fy  : [4x1] tire longitudinal/lateral forces, N
% Vsx,Vsy : [4x1] longitudinal/lateral sliding velocities, m/s
% dt      : sample time, s
%
% E_long_J = integral(sum(|Fx .* Vsx|) dt)
% E_lat_J  = integral(sum(|Fy .* Vsy|) dt)
% =========================================================================

    persistent E_long_acc E_lat_acc

    if isempty(E_long_acc) || double(is_reset(1)) > 0.5
        E_long_acc = 0.0;
        E_lat_acc  = 0.0;
    end

    Fx_vec  = double(reshape(Fx,  4, 1));
    Fy_vec  = double(reshape(Fy,  4, 1));
    Vsx_vec = double(reshape(Vsx, 4, 1));
    Vsy_vec = double(reshape(Vsy, 4, 1));

    dt_in = double(dt(1));
    if isnan(dt_in) || isinf(dt_in) || dt_in <= 1e-6
        dt_in = 0.01;
    end

    for i = 1:4
        if isnan(Fx_vec(i)) || isinf(Fx_vec(i)), Fx_vec(i) = 0.0; end
        if isnan(Fy_vec(i)) || isinf(Fy_vec(i)), Fy_vec(i) = 0.0; end
        if isnan(Vsx_vec(i)) || isinf(Vsx_vec(i)), Vsx_vec(i) = 0.0; end
        if isnan(Vsy_vec(i)) || isinf(Vsy_vec(i)), Vsy_vec(i) = 0.0; end
    end

    P_long_W = sum(abs(Fx_vec .* Vsx_vec));
    P_lat_W  = sum(abs(Fy_vec .* Vsy_vec));

    E_long_acc = E_long_acc + P_long_W * dt_in;
    E_lat_acc  = E_lat_acc  + P_lat_W  * dt_in;

    E_long_J = E_long_acc;
    E_lat_J  = E_lat_acc;
    E_slip_J = E_long_acc + E_lat_acc;

    E_slip_kWh = E_slip_J / 3.6e6;
end

== matlab function PGA_MPC_MODEL/Subsystem1/MATLAB Function22 ==
  data: Fx_fr input; Px_fr output; Fy_fr input; Sx_fr input; Sy_fr input; Vx input; Vy input; r input; delta_f input; lf input; twf input; Py_fr output
function [Px_fr, Py_fr] = Cal_Power_FR(Fx_fr, Fy_fr, Sx_fr, Sy_fr, Vx, Vy, r, delta_f, lf, twf)
% Cal_Power_FR - 右前轮横纵向滑移功耗计算
% 注意：运动学计算中的符号与左轮不同

    % 1. 重新计算轮心纵向速度 V_long
    % 运动学：右前轮位置 (+lf, -twf/2 => 右侧通常定义为y轴负方向或正方向，此处依据您之前的代码逻辑)
    % 依据之前的逻辑：右轮横摆分量是 Vx + r*(twf/2)
    V_cx = Vx + r * (twf / 2); 
    V_cy = Vy + r * lf;

    % 坐标旋转
    cos_d = cos(delta_f);
    sin_d = sin(delta_f);
    
    V_long = V_cx * cos_d + V_cy * sin_d;
    V_long_abs = max(abs(V_long), 1.0);

    % 2. 纵向滑移功耗
    Px_fr = abs(Fx_fr * (Sx_fr * V_long_abs));

    % 3. 横向滑移功耗
    Py_fr = abs(Fy_fr * (Sy_fr * V_long_abs));

end

== matlab function PGA_MPC_MODEL/Subsystem1/MATLAB Function24 ==
  data: Fx_rl input; Px_rl output; Fy_rl input; Sx_rl input; Sy_rl input; Vx input; Vy input; r input; lr input; twr input; Py_rl output
function [Px_rl, Py_rl] = Cal_Power_RL(Fx_rl, Fy_rl, Sx_rl, Sy_rl, Vx, Vy, r, lr, twr)
% Cal_Power_RL - 左后轮横纵向滑移功耗计算
% 后轮无转向角 delta，故 V_long 直接等于 V_cx

    % 1. 重新计算轮心纵向速度 V_long
    % 运动学：左后轮位置 (-lr, +twr/2)
    % 左轮：Vx - r * (twr/2)
    V_long = Vx - r * (twr / 2);
    
    % 后轮无转向，无需坐标旋转，V_long 即为轮心纵向速度
    V_long_abs = max(abs(V_long), 1.0);

    % 2. 纵向滑移功耗
    Px_rl = abs(Fx_rl * (Sx_rl * V_long_abs));

    % 3. 横向滑移功耗
    Py_rl = abs(Fy_rl * (Sy_rl * V_long_abs));

end

== matlab function PGA_MPC_MODEL/Subsystem1/MATLAB Function25 ==
  data: Fx_rr input; Px_rr output; Fy_rr input; Sx_rr input; Sy_rr input; Vx input; Vy input; r input; lr input; twr input; Py_rr output
function [Px_rr, Py_rr] = Cal_Power_RR(Fx_rr, Fy_rr, Sx_rr, Sy_rr, Vx, Vy, r, lr, twr)
% Cal_Power_RR - 右后轮横纵向滑移功耗计算

    % 1. 重新计算轮心纵向速度 V_long
    % 运动学：右后轮位置 (-lr, -twr/2)
    % 右轮：Vx + r * (twr/2)
    V_long = Vx + r * (twr / 2);
    
    V_long_abs = max(abs(V_long), 1.0);

    % 2. 纵向滑移功耗
    Px_rr = abs(Fx_rr * (Sx_rr * V_long_abs));

    % 3. 横向滑移功耗
    Py_rr = abs(Fy_rr * (Sy_rr * V_long_abs));

end

== matlab function PGA_MPC_MODEL/Subsystem1/MATLAB Function26 ==
  data: Sx_vec input; Sx_abs_vec output; Fx_vec input; Fy_vec input; Fz_vec input; Mu_in input; Sx_max output; Sx_rms output; Eta_vec output; Eta_max output; Eta_rms output; Debug_Info output
function [Sx_abs_vec, Sx_max, Sx_rms, Eta_vec, Eta_max, Eta_rms, Debug_Info] = ...
    Calc_Slip_And_TireUtilization_Vec(Sx_vec, Fx_vec, Fy_vec, Fz_vec, Mu_in)
%#codegen
% =========================================================================
% Calc_Slip_And_TireUtilization_Vec
%
% 输入（推荐全部为 4x1 列向量）：
%   Sx_vec = [Sx_fl; Sx_fr; Sx_rl; Sx_rr]
%   Fx_vec = [Fx_fl; Fx_fr; Fx_rl; Fx_rr]
%   Fy_vec = [Fy_fl; Fy_fr; Fy_rl; Fy_rr]
%   Fz_vec = [Fz_fl; Fz_fr; Fz_rl; Fz_rr]
%   Mu_in  = 当前路面附着系数
%
% 输出：
%   Sx_abs_vec : 四轮绝对纵向滑移率 [4x1]
%   Sx_max     : 四轮最大绝对纵向滑移率
%   Sx_rms     : 四轮纵向滑移率 RMS
%   Eta_vec    : 四轮附着利用率 [4x1]
%   Eta_max    : 四轮最大附着利用率
%   Eta_rms    : 四轮附着利用率 RMS
%   Debug_Info : 调试输出 [6x1]
%
% 公式：
%   Sx_max(t) = max_i |Sx_i(t)|
%   Sx_rms(t) = sqrt( (1/4) * sum_i Sx_i(t)^2 )
%   Eta_i(t)  = sqrt( (Fx_i/(mu*Fz_i))^2 + (Fy_i/(mu*Fz_i))^2 )
% =========================================================================

%% 1) 输入整理与保护
% 强制转成 4x1 列向量（Simulink 中请把输入维度直接设成 [4 1]）
Sx = reshape(double(Sx_vec), 4, 1);
Fx = reshape(double(Fx_vec), 4, 1);
Fy = reshape(double(Fy_vec), 4, 1);
Fz = reshape(double(Fz_vec), 4, 1);

% NaN / Inf 保护
for i = 1:4
    if isnan(Sx(i)) || isinf(Sx(i))
        Sx(i) = 0.0;
    end
    if isnan(Fx(i)) || isinf(Fx(i))
        Fx(i) = 0.0;
    end
    if isnan(Fy(i)) || isinf(Fy(i))
        Fy(i) = 0.0;
    end
    if isnan(Fz(i)) || isinf(Fz(i))
        Fz(i) = 0.0;
    end
end

Mu_safe = double(Mu_in(1));
if isnan(Mu_safe) || isinf(Mu_safe)
    Mu_safe = 0.85;
end
Mu_safe = max(0.05, min(Mu_safe, 1.20));

% 垂向载荷保护，避免除零
Fz_min = 100.0;
for i = 1:4
    Fz(i) = max(abs(Fz(i)), Fz_min);
end

eps_den = 1e-6;

%% 2) 四轮纵向滑移率综合指标
Sx_abs_vec = abs(Sx);

Sx_max = max(Sx_abs_vec);

Sx_rms = sqrt(0.25 * sum(Sx.^2));

%% 3) 四轮附着利用率 Eta_i(t)
Eta_vec = zeros(4,1);

for i = 1:4
    den_i = Mu_safe * Fz(i) + eps_den;
    Eta_vec(i) = sqrt((Fx(i)/den_i)^2 + (Fy(i)/den_i)^2);
end

Eta_max = max(Eta_vec);

Eta_rms = sqrt(0.25 * sum(Eta_vec.^2));

%% 4) Debug 输出
% [1] Sx_max
% [2] Sx_rms
% [3] Eta_max
% [4] Eta_rms
% [5] Mu_safe
% [6] min(Fz)
Debug_Info = [Sx_max; Sx_rms; Eta_max; Eta_rms; Mu_safe; min(Fz)];

end

== matlab function PGA_MPC_MODEL/Subsystem1/MATLAB Function27 ==
  data: Sx_rms input; I_Sx output; Station_m input; I_Sx_norm output; I_Debug output
function [I_Sx, I_Sx_norm, I_Debug] = Calc_Cumulative_Slip_Intensity(Sx_rms, Station_m)
%#codegen
% =========================================================================
% Online cumulative longitudinal slip intensity:
%   I_Sx(s) = integral_0^s Sx_rms^2(xi) dxi
% =========================================================================

persistent I_prev
persistent S_prev
persistent sx2_prev
persistent initialized

if isempty(initialized)
    I_prev = 0.0;
    S_prev = 0.0;
    sx2_prev = 0.0;
    initialized = false;
end

sx = double(Sx_rms(1));
if isnan(sx) || isinf(sx)
    sx = 0.0;
end
sx = abs(sx);

S_now = double(Station_m(1));
if isnan(S_now) || isinf(S_now)
    S_now = S_prev;
end

% 第一次运行，或者 Station 回到起点/发生倒退时，自动清零
if (~initialized) || (S_now < S_prev)
    I_prev = 0.0;
    S_prev = S_now;
    sx2_prev = sx * sx;
    initialized = true;
end

ds = S_now - S_prev;

if isnan(ds) || isinf(ds) || ds < 0.0
    ds = 0.0;
end

% 一般你的 Station 每步约 0.009 m，这里只是防异常跳点
ds_max = 20.0;
if ds > ds_max
    ds = ds_max;
end

sx2_now = sx * sx;

I_now = I_prev + 0.5 * (sx2_prev + sx2_now) * ds;

distance_safe = max(S_now, 1e-6);
I_norm_now = I_now / distance_safe;

I_prev = I_now;
S_prev = S_now;
sx2_prev = sx2_now;

I_Sx = I_now;
I_Sx_norm = I_norm_now;

% [1] I_Sx
% [2] I_Sx_norm
% [3] ds
% [4] input Sx_rms
% [5] Station_m
I_Debug = [I_Sx; I_Sx_norm; ds; sx; S_now];

end

== matlab function PGA_MPC_MODEL/Subsystem1/MATLAB Function20 ==
  data: Fx_fl input; Td output; Fx_fr input; Fx_rl input; Fx_rr input; r_e input; T_fl output; T_fr output; T_rl output; T_rr output
function[Td,T_fl,T_fr,T_rl,T_rr]  = calc_total_demand_torque(Fx_fl, Fx_fr, Fx_rl, Fx_rr, r_e)
% 计算总需求转矩Td
% 输入参数：
%   Fx_fl, Fx_fr, Fx_rl, Fx_rr: 四个车轮的纵向力 (N)，驱动为正，制动为负
%   r_e: 轮胎有效半径 (m)
% 输出参数：
%   Td: 总需求转矩 (Nm)

% 计算总纵向力
F_x_total = Fx_fl + Fx_fr + Fx_rl + Fx_rr;

% 总需求转矩 = 总纵向力 × 轮胎有效半径
T_fl = Fx_fl* r_e;
T_fr = Fx_fr* r_e;
T_rl = Fx_rl* r_e;
T_rr = Fx_rr* r_e;
Td = F_x_total * r_e;

% 数值稳定性处理（可选，若需避免极端值）
Td = real(Td);
end
